simulink subsystem "driver_request_old"  (R2022a)
settings: Solver=VariableStepAuto  StartTime=0.0  StopTime=10.0  RelTol=1e-3
settings Model: Creator=jutri  LastModifiedBy=Usuario
settings ModelReferenceCC: EnableRefExpFcnMdlSchedulingChecks=off
settings RTWCC: Description=Generic Real-Time Target  GPUComputeCapability=5.0

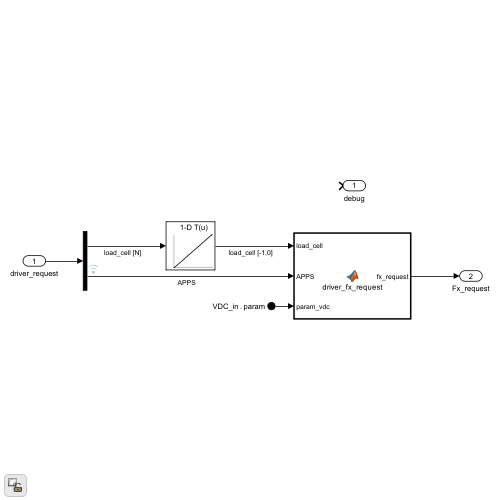
[thumbnail: Simulink's stored preview of the top-level diagram]
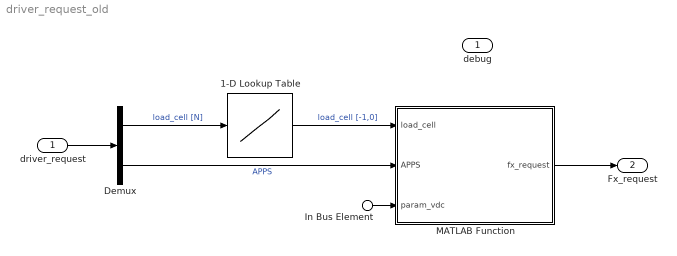
== system driver_request_old ==
  driver_request : Inport
  In Bus Element : Inport  Port=2  PortName=VDC_in  Element=param
  1-D Lookup Table : Lookup_n-D  NumberOfTableDimensions=1  BreakpointsForDimension1=[0;10;390;400]  Table=[0;0;1;1]  InternalRulePriority=Speed  RndMeth=Simplest
  Demux : Demux  Outputs=2
  MATLAB Function : MATLAB Function  TreatAsAtomicUnit=on
  debug : Outport
  Fx_request : Outport  Port=2
  wires:
  driver_request/1 -> Demux/1
  Demux/1 -> 1-D Lookup Table/1  "load_cell [N]"
  Demux/2 -> MATLAB Function/2(APPS)  "APPS"
  MATLAB Function/1(fx_request) -> Fx_request/1
  In Bus Element/1 -> MATLAB Function/3(param_vdc)
  1-D Lookup Table/1 -> MATLAB Function/1(load_cell)  "load_cell [-1,0]"

== matlab function driver_request_old/MATLAB Function ==
  data: load_cell input; fx_request output; APPS input; param_vdc input
function fx_request = driver_fx_request(load_cell, APPS, param_vdc)

% Comanda normalizada a [-1,1]
cmd_pos = sum(param_vdc.torque_limit_positive)*param_vdc.gear_ratio/param_vdc.rdyn*APPS;
cmd_neg = sum(param_vdc.torque_limit_negative)*param_vdc.gear_ratio/param_vdc.rdyn*load_cell;

% Salida: fx total [N]
fx_request = cmd_neg + cmd_pos;
